simulink model "SimpleTractionModel"  (R2014a)
settings: Solver=ode3  StartTime=0.0  StopTime=30  RelTol=1e-3
values from neighbouring files (symbols this model uses):
  y = linspace(1,100)    [DataLoggerCode.m]
undefined symbols (not defined in the file or in its folder): fdesignblkfcn, gcbh
libraries: simulink x6, Solver_SF x1
settings Model: Creator=zierdt.1  LastModifiedBy=zierdt.1

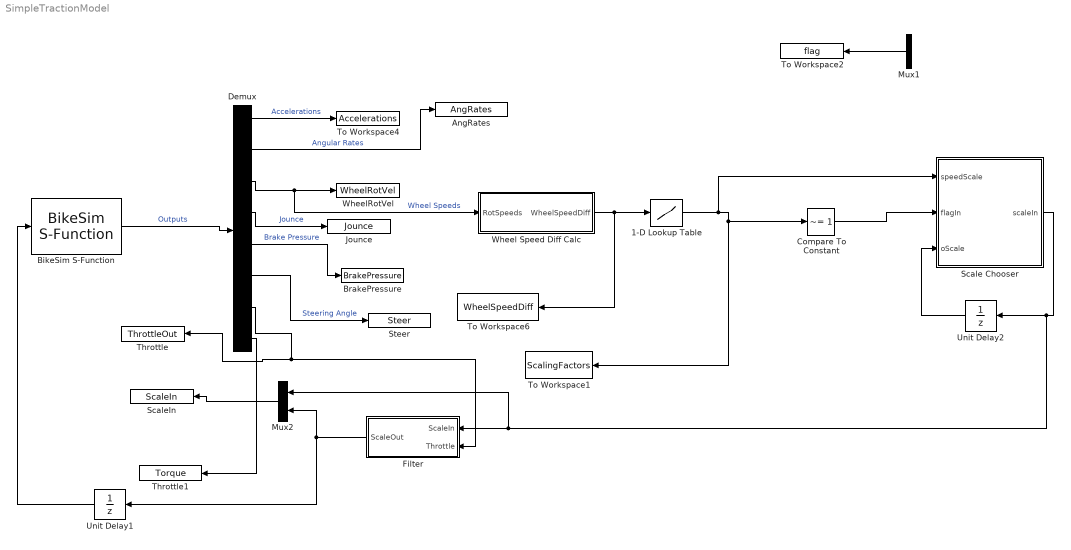
== system SimpleTractionModel ==
  1-D Lookup Table : Lookup_n-D  NumberOfTableDimensions=1  BreakpointsForDimension1=y  Table=[1.0000,0.9909,0.9818,0.9727,0.9636,0.9545,0.9455,0.9364,0.9273,0.9182,0.9091,0.9000,0.8909,0.8818,0.8727,0.8636,0.8545,0.8455,0.8364,0.8273,0.8182,0.8091,0.8000,0.7909,0.7818,0.7727,0.7636,0.7545,0.7455,0.7364,0.7273,0.7182,0.7091,0.7000,0.6909,0.6818,0.6727, 0.6636,0.6545,0.6455,0.6364,0.6273,0.6182,0.6091,0.6000,0.5909,0.5818,0.5727,0.5636,0.5545,0.5455,0.5364,0.5273,0.5182,0.5091,0.50, 0.4909,0.4818,0.4727,0.4636,0.4545,0.4455,0.4364,0.4273,0.4182,0.4091,0.40,0.3909,0.3818,0.3727,0.3636,0.3545,0.3455,0.3364,0.3273,0.3182,0.3091,0.3000,0.2909,0.2818,0.2727,0.2636,0.2545,0.2455,0.2364,0.2273 ,0.2182,0.2091,0.20,0.1909,0.1818,0.1727,0.1636,0.1545,0.1455,0.1364,0.1273,0.1182,0.1091,0.1000]  InterpMethod=Flat  ExtrapMethod=Clip  UseLastTableValue=on  InternalRulePriority=Speed  RndMeth=Simplest  InputSameDT=on
  AngRates : ToWorkspace  VariableName=AngRates  SaveFormat=Timeseries  SampleTime=-1
  BikeSim S-Function : Solver_SF/BikeSim S-Function  Priority=1  VehicleCode=fixed_caster  SIMFILE=simfile.sim
      settings: AttributesFormatString=Vehicle Code: %<VehicleCode>
  BrakePressure : ToWorkspace  VariableName=BrakePressure  SaveFormat=Timeseries  SampleTime=-1
  Compare To Constant : simulink/Logic and Bit Operations/Compare To Constant  relop=~=  const=1  OutDataTypeStr=boolean
  Demux : Demux  Outputs=[3 2 2 2 2 1 1 3]
  Filter : Subsystem
  Jounce : ToWorkspace  VariableName=Jounce  SaveFormat=Timeseries  SampleTime=-1
  Mux1 : Mux  Inputs=2
  Mux2 : Mux  Inputs=2
  Scale Chooser : MATLAB Function  TreatAsAtomicUnit=on
  ScaleIn : ToWorkspace  VariableName=ScaleIn  SaveFormat=Timeseries  SampleTime=-1
  Steer : ToWorkspace  VariableName=Steer  SaveFormat=Timeseries  SampleTime=-1
  Throttle : ToWorkspace  VariableName=ThrottleOut  SaveFormat=Timeseries  SampleTime=-1
  Throttle1 : ToWorkspace  VariableName=Torque  SaveFormat=Timeseries  SampleTime=-1
  To Workspace1 : ToWorkspace  VariableName=ScalingFactors  SaveFormat=Timeseries  SampleTime=-1
  To Workspace2 : ToWorkspace  VariableName=flag  SaveFormat=Timeseries  SampleTime=-1
  To Workspace4 : ToWorkspace  VariableName=Accelerations  SaveFormat=Timeseries  SampleTime=-1
  To Workspace6 : ToWorkspace  VariableName=WheelSpeedDiff  SaveFormat=Timeseries  SampleTime=-1
  Unit Delay1 : UnitDelay  SampleTime=-1
  Unit Delay2 : UnitDelay  SampleTime=-1
  Wheel Speed Diff Calc : Subsystem
  WheelRotVel : ToWorkspace  VariableName=WheelRotVel  SaveFormat=Timeseries  SampleTime=-1
  wires:
  Demux/1 -> To Workspace4/1  "Accelerations"
  Demux/3 -> WheelRotVel/1, Wheel Speed Diff Calc/1(RotSpeeds)  "Wheel Speeds"
  Demux/4 -> Jounce/1  "Jounce"
  Demux/5 -> BrakePressure/1  "Brake Pressure"
  Demux/6 -> Steer/1  "Steering Angle"
  BikeSim S-Function/1 -> Demux/1  "Outputs"
  Demux/7 -> Throttle/1, Filter/2(Throttle)
  Demux/2 -> AngRates/1  "Angular Rates"
  Wheel Speed Diff Calc/1(WheelSpeedDiff) -> To Workspace6/1, 1-D Lookup Table/1
  Mux2/1 -> ScaleIn/1
  Demux/8 -> Throttle1/1
  Filter/1(ScaleOut) -> Mux2/2, Unit Delay1/1
  Mux1/1 -> To Workspace2/1
  Unit Delay1/1 -> BikeSim S-Function/1
  1-D Lookup Table/1 -> Scale Chooser/1(speedScale), Compare To Constant/1, To Workspace1/1
  Scale Chooser/1(scaleIn) -> Mux2/1, Filter/1(ScaleIn), Unit Delay2/1
  Unit Delay2/1 -> Scale Chooser/3(oScale)
  Compare To Constant/1 -> Scale Chooser/2(flagIn)

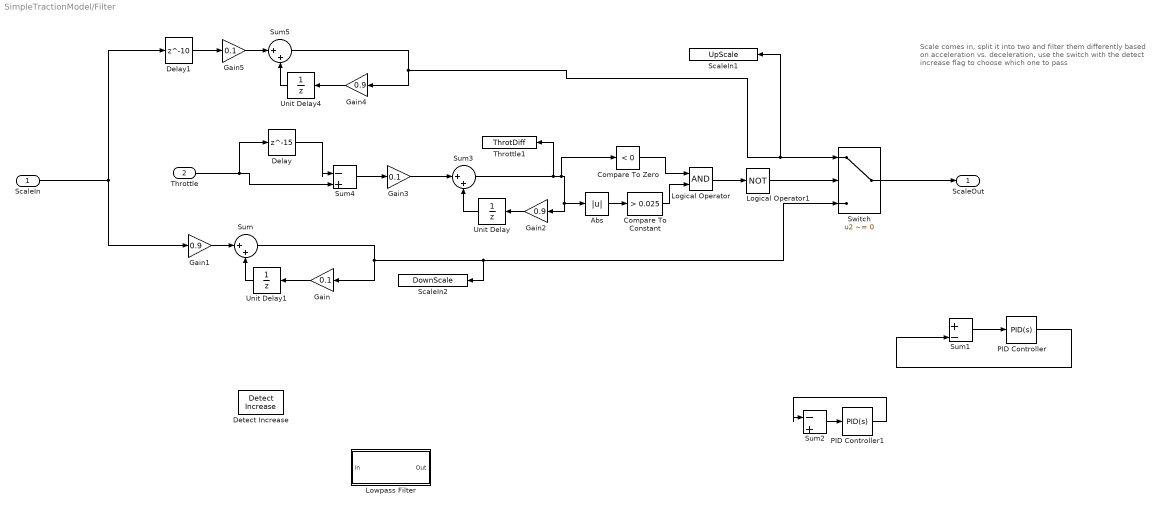
== system SimpleTractionModel/Filter ==
  note: Scale comes in, split it into two and filter them differently
      | based on acceleration vs. deceleration, use the switch with
      | the detect increase flag to choose which one to pass
  ScaleIn : Inport
  Throttle : Inport  Port=2
  Abs : Abs
  Compare To Constant : simulink/Logic and Bit Operations/Compare To Constant  relop=>  const=0.025  OutDataTypeStr=boolean
  Compare To Zero : simulink/Logic and Bit Operations/Compare To Zero  relop=<  OutDataTypeStr=boolean
  Delay : Delay  DelayLength=15
  Delay1 : Delay  DelayLength=10
  Detect Increase : simulink/Logic and Bit Operations/Detect Increase  vinit=0.0  InputProcessing=Inherited  OutDataTypeStr=uint8
  Gain : Gain  Gain=0.1
  Gain1 : Gain  Gain=0.9
  Gain2 : Gain  Gain=0.9
  Gain3 : Gain  Gain=0.1
  Gain4 : Gain  Gain=0.9
  Gain5 : Gain  Gain=0.1
  Logical Operator : Logic  AllPortsSameDT=off  OutDataTypeStr=boolean
  Logical Operator1 : Logic  Operator=NOT  AllPortsSameDT=off  OutDataTypeStr=boolean
  Lowpass Filter : Subsystem  DialogController=fdesignblkfcn  InitFcn=fdesignblkfcn(gcbh, {'InitFcn'});  mask(Lowpass Filter){}
      mask help: Design a lowpass filter
      settings: CopyFcn=fdesignblkfcn(gcbh, {'CopyFcn'});
      mask Help: helpview(mapfilelocation('dsp'), 'dsplowpassfilter');
      mask Display: disp('Lowpass')
  PID Controller : simulink/Continuous/PID Controller  Controller=PID  TimeDomain=Continuous-time  SampleTime=1  IntegratorMethod=Forward Euler  FilterMethod=Forward Euler  Form=Parallel  P=0.01  I=0.4  D=0.01  N=100  InitialConditionSource=internal  InitialConditionForIntegrator=1  InitialConditionForFilter=0  ExternalReset=none  LimitOutput=off  UpperSaturationLimit=inf  LowerSaturationLimit=-inf  LinearizeAsGain=on  AntiWindupMode=none  Kb=1  TrackingMode=off  Kt=1  PParamMin=[]  PParamMax=[]  IParamMin=[]  IParamMax=[]  DParamMin=[]  DParamMax=[]  NParamMin=[]  NParamMax=[]  KbParamMin=[]  KbParamMax=[]  KtParamMin=[]  KtParamMax=[]  POutMin=[]  POutMax=[]  IOutMin=[]  IOutMax=[]  DOutMin=[]  DOutMax=[]  NOutMin=[]  NOutMax=[]  KbOutMin=[]  KbOutMax=[]  KtOutMin=[]  KtOutMax=[]  IntegratorOutMin=[]  IntegratorOutMax=[]  FilterOutMin=[]  FilterOutMax=[]  SumOutMin=[]  SumOutMax=[]  SumI1OutMin=[]  SumI1OutMax=[]  SumI2OutMin=[]  SumI2OutMax=[]  SumI3OutMin=[]  SumI3OutMax=[]  SumDOutMin=[]  SumDOutMax=[]  SaturationOutMin=[]  SaturationOutMax=[]  IntegratorContinuousStateAttributes=''  IntegratorStateMustResolveToSignalObject=off  IntegratorRTWStateStorageClass=Auto  FilterContinuousStateAttributes=''  FilterStateMustResolveToSignalObject=off  FilterRTWStateStorageClass=Auto
  PID Controller1 : simulink/Continuous/PID Controller  Controller=PID  TimeDomain=Continuous-time  SampleTime=1  IntegratorMethod=Forward Euler  FilterMethod=Forward Euler  Form=Parallel  P=0  I=1.90546071796325  D=0  N=100  InitialConditionSource=internal  InitialConditionForIntegrator=1  InitialConditionForFilter=0  ExternalReset=none  LimitOutput=off  UpperSaturationLimit=inf  LowerSaturationLimit=-inf  LinearizeAsGain=on  AntiWindupMode=none  Kb=1  TrackingMode=off  Kt=1  PParamMin=[]  PParamMax=[]  IParamMin=[]  IParamMax=[]  DParamMin=[]  DParamMax=[]  NParamMin=[]  NParamMax=[]  KbParamMin=[]  KbParamMax=[]  KtParamMin=[]  KtParamMax=[]  POutMin=[]  POutMax=[]  IOutMin=[]  IOutMax=[]  DOutMin=[]  DOutMax=[]  NOutMin=[]  NOutMax=[]  KbOutMin=[]  KbOutMax=[]  KtOutMin=[]  KtOutMax=[]  IntegratorOutMin=[]  IntegratorOutMax=[]  FilterOutMin=[]  FilterOutMax=[]  SumOutMin=[]  SumOutMax=[]  SumI1OutMin=[]  SumI1OutMax=[]  SumI2OutMin=[]  SumI2OutMax=[]  SumI3OutMin=[]  SumI3OutMax=[]  SumDOutMin=[]  SumDOutMax=[]  SaturationOutMin=[]  SaturationOutMax=[]  IntegratorContinuousStateAttributes=''  IntegratorStateMustResolveToSignalObject=off  IntegratorRTWStateStorageClass=Auto  FilterContinuousStateAttributes=''  FilterStateMustResolveToSignalObject=off  FilterRTWStateStorageClass=Auto
  ScaleIn1 : ToWorkspace  VariableName=UpScale  SaveFormat=Timeseries  SampleTime=-1
  ScaleIn2 : ToWorkspace  VariableName=DownScale  SaveFormat=Timeseries  SampleTime=-1
  Sum : Sum  Inputs=|++
  Sum1 : Sum  Inputs=|+-
  Sum2 : Sum  Inputs=|-+
  Sum3 : Sum  Inputs=|++
  Sum4 : Sum  Inputs=|-+
  Sum5 : Sum  Inputs=|++
  Switch : Switch  Criteria=u2 ~= 0  OutMin=[0.1]  OutMax=[1]
  Throttle1 : ToWorkspace  VariableName=ThrotDiff  SaveFormat=Timeseries  SampleTime=-1
  Unit Delay : UnitDelay  SampleTime=-1
  Unit Delay1 : UnitDelay  SampleTime=-1
  Unit Delay4 : UnitDelay  SampleTime=-1
  ScaleOut : Outport
  wires:
  Gain1/1 -> Sum/1
  Gain/1 -> Unit Delay1/1
  Sum1/1 -> PID Controller/1
  Sum2/1 -> PID Controller1/1
  Gain3/1 -> Sum3/1
  Gain2/1 -> Unit Delay/1
  Sum3/1 -> Throttle1/1, Compare To Zero/1, Abs/1, Gain2/1
  PID Controller1/1 -> Sum2/1
  Unit Delay1/1 -> Sum/2
  Unit Delay/1 -> Sum3/2
  Sum/1 -> Gain/1, ScaleIn2/1, Switch/3
  Sum5/1 -> ScaleIn1/1, Switch/1, Gain4/1
  PID Controller/1 -> Sum1/2
  Throttle/1 -> Delay/1, Sum4/2
  Sum4/1 -> Gain3/1
  Gain5/1 -> Sum5/1
  Gain4/1 -> Unit Delay4/1
  Unit Delay4/1 -> Sum5/2
  ScaleIn/1 -> Gain1/1, Delay1/1
  Delay/1 -> Sum4/1
  Delay1/1 -> Gain5/1
  Abs/1 -> Compare To Constant/1
  Compare To Zero/1 -> Logical Operator/1
  Compare To Constant/1 -> Logical Operator/2
  Logical Operator/1 -> Logical Operator1/1
  Logical Operator1/1 -> Switch/2
  Switch/1 -> ScaleOut/1

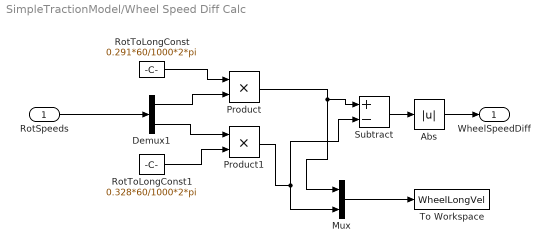
== system SimpleTractionModel/Wheel Speed Diff Calc ==
  RotSpeeds : Inport
  Abs : Abs
  Demux1 : Demux  Outputs=2
  Mux : Mux  Inputs=2
  Product : Product
  Product1 : Product
  RotToLongConst : Constant  Value=0.291*60/1000*2*pi
  RotToLongConst1 : Constant  Value=0.328*60/1000*2*pi
  Subtract : Sum  Inputs=+-
  To Workspace : ToWorkspace  VariableName=WheelLongVel  SaveFormat=Timeseries  SampleTime=-1
  WheelSpeedDiff : Outport
  wires:
  RotSpeeds/1 -> Demux1/1
  Demux1/1 -> Product/2
  Demux1/2 -> Product1/1
  RotToLongConst/1 -> Product/1
  RotToLongConst1/1 -> Product1/2
  Product/1 -> Subtract/1, Mux/1
  Product1/1 -> Subtract/2, Mux/2
  Subtract/1 -> Abs/1
  Abs/1 -> WheelSpeedDiff/1
  Mux/1 -> To Workspace/1

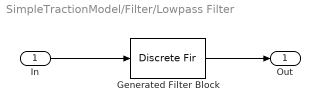
== system SimpleTractionModel/Filter/Lowpass Filter ==
  In : Inport
  Generated Filter Block : DiscreteFir  Tag=BlockMethodSubSystem  Coefficients=[-0.0024228738523269142 -0.002083244982079274 0.0067703446401187091 0.016731945423489058 0.011117076081077608 -0.0062311454141445394 -0.008401617186026911 0.0092567976151380175 0.012982883808855752 -0.010121234703278968 -0.018273518733782485 0.011431962071777957 0.02617588858040763 -0.012489027835322923 -0.037996623145463579 0.013388945199366963 0.058155465814729891 -0.014048043515808939 -0.10272466857882172 0.014462275771238358 0.31716649721769491 0.48538764678732504 0.31716649721769491 0.014462275771238358 -0.10272466857882172 -0.014048043515808939 0.058155465814729891 0.013388945199366963 -0.037996623145463579 -0.012489027835322923 0.02617588858040763 0.011431962071777957 -0.018273518733782485 -0.010121234703278968 0.012982883808855752 0.0092567976151380175 -0.008401617186026911 -0.0062311454141445394 0.011117076081077608 0.016731945423489058 0.0067703446401187091 -0.002083244982079274 -0.0024228738523269142]  InputProcessing=Columns as channels (frame based)
  Out : Outport
  wires:
  In/1 -> Generated Filter Block/1
  Generated Filter Block/1 -> Out/1

== matlab function SimpleTractionModel/Scale Chooser ==
  data: scaleIn output; speedScale input; flagIn input; oScale input
function scaleIn = fcn(speedScale, flagIn,oScale)
if flagIn==0 %flag is 0 to start, meaning no scaling has occurred
    if oScale==0
        scaleIn=1;
    else
        scaleIn=oScale;
    end
else %Throttle has been scaled
    if flagIn==1 && oScale~=speedScale %speed scaling occurred, scale changed
        scaleIn=1/oScale*speedScale; %re-scale throttle
    else %scaling occurred, scale didn't change, indicator(s) still being thrown
        scaleIn=1;
    end       
end
